simulink model "SSD_Pro"  (R2025b)
settings: Solver=FixedStepDiscrete  StartTime=0.0  StopTime=200  FixedStep=0.1  RelTol=1e-3
InitFcn:
  | addpath('C:\Users\dhanv\OneDrive\Desktop\ByteForce-Simulation\ByteForce-Simulation\simulink'); rehash;
undefined symbols (not defined in the file or in its folder): computeEventCode, DiscIntNeverNeededParam, simulinkPublishStep
libraries: simulink x6
settings Model: DataTypeOverride=Double  Creator=dhanv  LastModifiedBy=dhanv

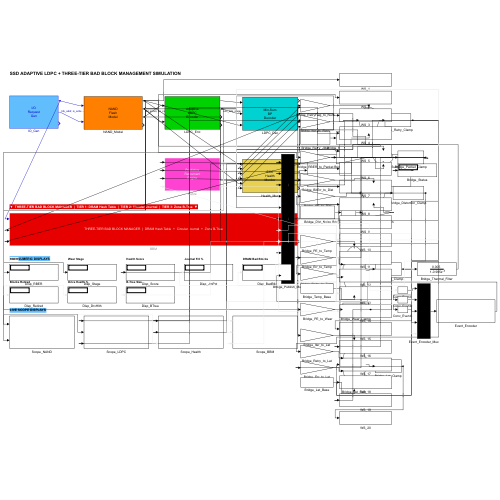
[thumbnail: Simulink's stored preview of the top-level diagram]
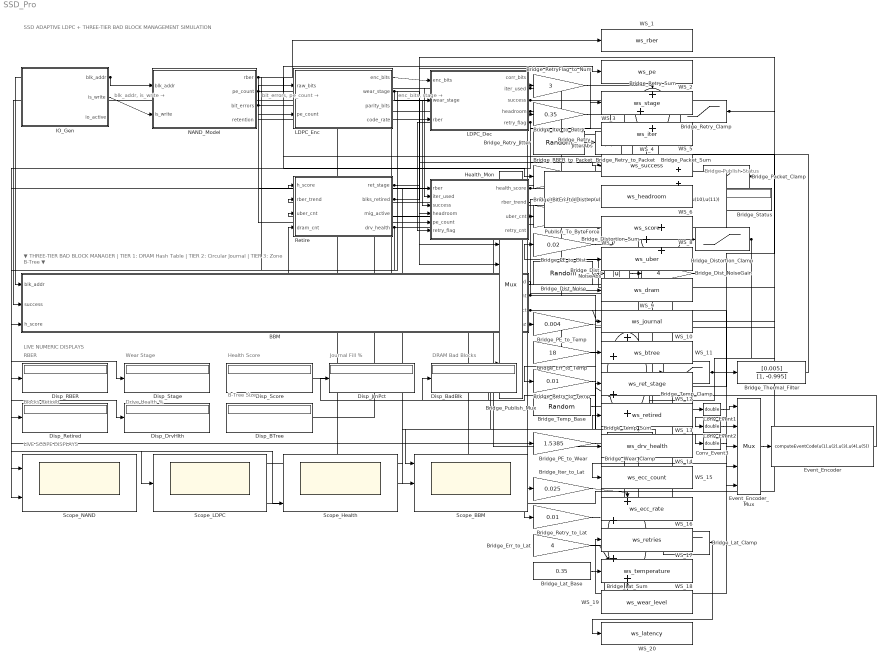
== system SSD_Pro ==
  note: Bridge Publish Status
  note: RBER
  note: Wear Stage
  note: Health Score
  note: Journal Fill %
  note: DRAM Bad Blocks
  note: Blocks Retired
  note: Drive Health %
  note: B-Tree Size
  note: blk_addr, is_write →
  note: bit_errors, pe_count →
  note: enc_bits, stage →
  note: SSD ADAPTIVE LDPC + THREE-TIER BAD BLOCK MANAGEMENT SIMULATION
  note: ▼ THREE-TIER BAD BLOCK MANAGER | TIER 1: DRAM Hash Table | TIER 2: Circular Journal | TIER 3: Zone B-Tree ▼
  note: LIVE NUMERIC DISPLAYS
  note: LIVE SCOPE DISPLAYS
  BBM : Subsystem
      mask Display: disp('THREE-TIER BAD BLOCK MANAGER  |  DRAM Hash Table  +  Circular Journal  +  Zone B-Tree')
  Bridge_BitErr_to_Dist : Gain  Gain=0.25
  Bridge_Dist_Noise : RandomNumber  Seed=9340  SampleTime=0.1
  Bridge_Dist_NoiseAbs : Abs  SaturateOnIntegerOverflow=off
  Bridge_Dist_NoiseGain : Gain  Gain=4
  Bridge_Distortion_Clamp : Saturate  UpperLimit=1e6  LowerLimit=0
  Bridge_Distortion_Sum : Sum  Inputs=+++
  Bridge_Err_to_Lat : Gain  Gain=4
  Bridge_Err_to_Temp : Gain  Gain=18
  Bridge_Iter_to_Lat : Gain  Gain=0.025
  Bridge_Iter_to_Retry : Gain  Gain=0.35
  Bridge_Lat_Base : Constant  Value=0.35
  Bridge_Lat_Clamp : Saturate  UpperLimit=20  LowerLimit=0.1
  Bridge_Lat_Sum : Sum  Inputs=++++
  Bridge_PE_to_Dist : Gain  Gain=0.02
  Bridge_PE_to_Temp : Gain  Gain=0.004
  Bridge_PE_to_Wear : Gain  Gain=1.5385
  Bridge_Packet_Clamp : Saturate  UpperLimit=1  LowerLimit=0
  Bridge_Packet_Sum : Sum
  Bridge_Publish_Mux : Mux  Inputs=11
  Bridge_RBER_to_Packet : Gain  Gain=4
  Bridge_RetryFlag_to_Num : Gain  Gain=3
  Bridge_Retry_Clamp : Saturate  UpperLimit=250  LowerLimit=0
  Bridge_Retry_Jitter : RandomNumber  Variance=4  Seed=8492  SampleTime=0.1
  Bridge_Retry_JitterAbs : Abs  SaturateOnIntegerOverflow=off
  Bridge_Retry_Sum : Sum  Inputs=+++
  Bridge_Retry_to_Lat : Gain  Gain=0.01
  Bridge_Retry_to_Packet : Gain  Gain=0.0015
  Bridge_Retry_to_Temp : Gain  Gain=0.01
  Bridge_Status : Display
  Bridge_Temp_Base : RandomNumber  Mean=30  Variance=25  Seed=6788  SampleTime=0.1
  Bridge_Temp_Clamp : Saturate  UpperLimit=95  LowerLimit=20
  Bridge_Temp_Sum : Sum  Inputs=++++
  Bridge_Thermal_Filter : DiscreteFilter  Numerator=[0.005]  Denominator=[1, -0.995]  SampleTime=0.1
  Bridge_Wear_Clamp : Saturate  UpperLimit=100  LowerLimit=0
  Conv_Event1 : DataTypeConversion  OutDataTypeStr=double  SaturateOnIntegerOverflow=off  RndMeth=Floor
  Conv_Event2 : DataTypeConversion  OutDataTypeStr=double  SaturateOnIntegerOverflow=off  RndMeth=Floor
  Conv_Event3 : DataTypeConversion  OutDataTypeStr=double  SaturateOnIntegerOverflow=off  RndMeth=Floor
  Disp_BTree : Display
  Disp_BadBlk : Display
  Disp_DrvHlth : Display
  Disp_JrnPct : Display
  Disp_RBER : Display
  Disp_Retired : Display
  Disp_Score : Display
  Disp_Stage : Display
  Event_Encoder : MATLABFcn  MATLABFcn=computeEventCode(u(1),u(2),u(3),u(4),u(5))
  Event_Encoder_Mux : Mux  Inputs=5
  Health_Mon : Subsystem
      mask Display: disp('ECC\nHealth\nMonitor')
  IO_Gen : Subsystem
      mask Display: disp('I/O\nRequest\nGen')
  LDPC_Dec : Subsystem
      mask Display: disp('Min-Sum\nBP\nDecoder')
  LDPC_Enc : Subsystem
      mask Display: disp('Adaptive\nLDPC\nEncoder')
  NAND_Model : Subsystem
      mask Display: disp('NAND\nFlash\nModel')
  Publish_To_ByteForce : MATLABFcn  MATLABFcn=simulinkPublishStep(u(1),u(2),u(3),u(4),u(5),u(6),u(7),u(8),u(9),u(10),u(11))
  Retire : Subsystem
      mask Display: disp('Predictive\nRetirement\nEngine')
  Scope_BBM : Scope  NumInputPorts=3
      settings: Title=Three-Tier BBM: DRAM Count | Journal % | B-Tree Size  YLabel=Count / %
  Scope_Health : Scope  NumInputPorts=3
      settings: Title=Block Health Score | UBER Count | Retirement Stage  YLabel=Value
  Scope_LDPC : Scope  NumInputPorts=3
      settings: Title=LDPC Decoder: Iterations | Success | Headroom %  YLabel=Value
  Scope_NAND : Scope  NumInputPorts=2
      settings: Title=NAND Degradation: RBER & PE Count  YLabel=Value
  WS_1 : ToWorkspace  VariableName=ws_rber  SaveFormat=Structure With Time  SampleTime=0.1
  WS_10 : ToWorkspace  VariableName=ws_journal  SaveFormat=Structure With Time  SampleTime=0.1
  WS_11 : ToWorkspace  VariableName=ws_btree  SaveFormat=Structure With Time  SampleTime=0.1
  WS_12 : ToWorkspace  VariableName=ws_ret_stage  SaveFormat=Structure With Time  SampleTime=0.1
  WS_13 : ToWorkspace  VariableName=ws_retired  SaveFormat=Structure With Time  SampleTime=0.1
  WS_14 : ToWorkspace  VariableName=ws_drv_health  SaveFormat=Structure With Time  SampleTime=0.1
  WS_15 : ToWorkspace  VariableName=ws_ecc_count  SaveFormat=Structure With Time  SampleTime=0.1
  WS_16 : ToWorkspace  VariableName=ws_ecc_rate  SaveFormat=Structure With Time  SampleTime=0.1
  WS_17 : ToWorkspace  VariableName=ws_retries  SaveFormat=Structure With Time  SampleTime=0.1
  WS_18 : ToWorkspace  VariableName=ws_temperature  SaveFormat=Structure With Time  SampleTime=0.1
  WS_19 : ToWorkspace  VariableName=ws_wear_level  SaveFormat=Structure With Time  SampleTime=0.1
  WS_2 : ToWorkspace  VariableName=ws_pe  SaveFormat=Structure With Time  SampleTime=0.1
  WS_20 : ToWorkspace  VariableName=ws_latency  SaveFormat=Structure With Time  SampleTime=0.1
  WS_3 : ToWorkspace  VariableName=ws_stage  SaveFormat=Structure With Time  SampleTime=0.1
  WS_4 : ToWorkspace  VariableName=ws_iter  SaveFormat=Structure With Time  SampleTime=0.1
  WS_5 : ToWorkspace  VariableName=ws_success  SaveFormat=Structure With Time  SampleTime=0.1
  WS_6 : ToWorkspace  VariableName=ws_headroom  SaveFormat=Structure With Time  SampleTime=0.1
  WS_7 : ToWorkspace  VariableName=ws_score  SaveFormat=Structure With Time  SampleTime=0.1
  WS_8 : ToWorkspace  VariableName=ws_uber  SaveFormat=Structure With Time  SampleTime=0.1
  WS_9 : ToWorkspace  VariableName=ws_dram  SaveFormat=Structure With Time  SampleTime=0.1
  wires:
  IO_Gen/1(blk_addr) -> NAND_Model/1(blk_addr), BBM/1(blk_addr)
  IO_Gen/2(is_write) -> NAND_Model/2(is_write)
  NAND_Model/3(bit_errors) -> LDPC_Enc/1(raw_bits), Bridge_BitErr_to_Dist/1
  NAND_Model/2(pe_count) -> LDPC_Enc/2(pe_count), Health_Mon/5(pe_count), Bridge_PE_to_Dist/1, Bridge_PE_to_Temp/1, Bridge_PE_to_Wear/1, Scope_NAND/2, WS_2/1
  LDPC_Enc/1(enc_bits) -> LDPC_Dec/1(enc_bits)
  LDPC_Enc/2(wear_stage) -> LDPC_Dec/2(wear_stage), Event_Encoder_Mux/4, Disp_Stage/1, WS_3/1
  NAND_Model/1(rber) -> LDPC_Dec/3(rber), Health_Mon/1(rber), Bridge_RBER_to_Packet/1, Disp_RBER/1, Scope_NAND/1, WS_1/1
  LDPC_Dec/2(iter_used) -> Health_Mon/2(iter_used), Bridge_Iter_to_Retry/1, Bridge_Iter_to_Lat/1, Scope_LDPC/1, WS_4/1
  LDPC_Dec/3(success) -> Health_Mon/3(success), BBM/2(success), Conv_Event2/1, Scope_LDPC/2, WS_5/1
  LDPC_Dec/4(headroom) -> Health_Mon/4(headroom), Scope_LDPC/3, WS_6/1
  LDPC_Dec/5(retry_flag) -> Health_Mon/6(retry_flag), Bridge_RetryFlag_to_Num/1, Conv_Event3/1
  Health_Mon/1(health_score) -> BBM/3(h_score), Retire/1(h_score), Disp_Score/1, Scope_Health/1, WS_7/1
  Health_Mon/2(rber_trend) -> Retire/2(rber_trend)
  Health_Mon/3(uber_cnt) -> Retire/3(uber_cnt), Bridge_Publish_Mux/9, Scope_Health/2, WS_8/1
  BBM/2(dram_cnt) -> Retire/4(dram_cnt), Bridge_Publish_Mux/7, Disp_BadBlk/1, Scope_BBM/1, WS_9/1
  Bridge_Retry_Jitter/1 -> Bridge_Retry_JitterAbs/1
  Bridge_RetryFlag_to_Num/1 -> Bridge_Retry_Sum/1
  Bridge_Iter_to_Retry/1 -> Bridge_Retry_Sum/2
  Bridge_Retry_JitterAbs/1 -> Bridge_Retry_Sum/3
  Bridge_Retry_Sum/1 -> Bridge_Retry_Clamp/1
  Bridge_Retry_Clamp/1 -> Bridge_Retry_to_Packet/1, Bridge_Retry_to_Temp/1, Bridge_Retry_to_Lat/1, Bridge_Publish_Mux/3, WS_17/1
  Bridge_RBER_to_Packet/1 -> Bridge_Packet_Sum/1
  Bridge_Retry_to_Packet/1 -> Bridge_Packet_Sum/2
  Bridge_Packet_Sum/1 -> Bridge_Packet_Clamp/1
  Bridge_Dist_Noise/1 -> Bridge_Dist_NoiseAbs/1
  Bridge_Dist_NoiseAbs/1 -> Bridge_Dist_NoiseGain/1
  Bridge_BitErr_to_Dist/1 -> Bridge_Distortion_Sum/1
  Bridge_PE_to_Dist/1 -> Bridge_Distortion_Sum/2
  Bridge_Dist_NoiseGain/1 -> Bridge_Distortion_Sum/3
  Bridge_Distortion_Sum/1 -> Bridge_Distortion_Clamp/1
  Bridge_Packet_Clamp/1 -> Bridge_Err_to_Temp/1, Bridge_Err_to_Lat/1, Bridge_Publish_Mux/2, WS_16/1
  Bridge_PE_to_Temp/1 -> Bridge_Temp_Sum/1
  Bridge_Err_to_Temp/1 -> Bridge_Temp_Sum/2
  Bridge_Retry_to_Temp/1 -> Bridge_Temp_Sum/3
  Bridge_Temp_Base/1 -> Bridge_Temp_Sum/4
  Bridge_Temp_Sum/1 -> Bridge_Temp_Clamp/1
  Bridge_PE_to_Wear/1 -> Bridge_Wear_Clamp/1
  Bridge_Iter_to_Lat/1 -> Bridge_Lat_Sum/1
  Bridge_Retry_to_Lat/1 -> Bridge_Lat_Sum/2
  Bridge_Err_to_Lat/1 -> Bridge_Lat_Sum/3
  Bridge_Lat_Base/1 -> Bridge_Lat_Sum/4
  Bridge_Lat_Sum/1 -> Bridge_Lat_Clamp/1
  Bridge_Temp_Clamp/1 -> Bridge_Thermal_Filter/1, WS_18/1
  BBM/1(is_bad) -> Conv_Event1/1
  Conv_Event1/1 -> Event_Encoder_Mux/1
  Conv_Event2/1 -> Event_Encoder_Mux/2
  Conv_Event3/1 -> Event_Encoder_Mux/3
  BBM/3(journal_pct) -> Event_Encoder_Mux/5, Bridge_Publish_Mux/8, Disp_JrnPct/1, Scope_BBM/2, WS_10/1
  Event_Encoder_Mux/1 -> Event_Encoder/1
  Event_Encoder/1 -> Bridge_Publish_Mux/11
  Bridge_Distortion_Clamp/1 -> Bridge_Publish_Mux/1, WS_15/1
  Bridge_Thermal_Filter/1 -> Bridge_Publish_Mux/4
  Bridge_Wear_Clamp/1 -> Bridge_Publish_Mux/5, WS_19/1
  Bridge_Lat_Clamp/1 -> Bridge_Publish_Mux/6, WS_20/1
  Retire/1(ret_stage) -> Bridge_Publish_Mux/10, Scope_Health/3, WS_12/1
  Bridge_Publish_Mux/1 -> Publish_To_ByteForce/1
  Publish_To_ByteForce/1 -> Bridge_Status/1
  Retire/2(blks_retired) -> Disp_Retired/1, WS_13/1
  Retire/4(drv_health) -> Disp_DrvHlth/1, WS_14/1
  BBM/4(btree_sz) -> Disp_BTree/1, Scope_BBM/3, WS_11/1

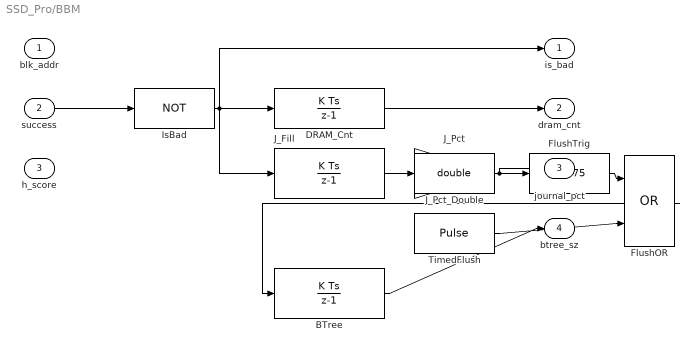
== system SSD_Pro/BBM ==
  blk_addr : Inport
  success : Inport  Port=2
  h_score : Inport  Port=3
  BTree : DiscreteIntegrator  SampleTime=0.1  UpperSaturationLimit=512  ICPrevOutput=DiscIntNeverNeededParam  ICPrevScaledInput=DiscIntNeverNeededParam
  DRAM_Cnt : DiscreteIntegrator  SampleTime=0.1  UpperSaturationLimit=512  ICPrevOutput=DiscIntNeverNeededParam  ICPrevScaledInput=DiscIntNeverNeededParam
  FlushOR : Logic  Operator=OR  AllPortsSameDT=off  OutDataTypeStr=boolean
  FlushTrig : simulink/Logic and Bit Operations/Compare To Constant  relop=>=  const=75  OutDataTypeStr=boolean
  IsBad : Logic  Operator=NOT  AllPortsSameDT=off  OutDataTypeStr=boolean
  J_Fill : DiscreteIntegrator  SampleTime=0.1  UpperSaturationLimit=64  LowerSaturationLimit=0  ICPrevOutput=DiscIntNeverNeededParam  ICPrevScaledInput=DiscIntNeverNeededParam
  J_Pct : Gain  Gain=1.5625
  J_Pct_Double : DataTypeConversion  OutDataTypeStr=double  RndMeth=Floor
  TimedFlush : DiscretePulseGenerator  PulseType=Time based  Period=15  PulseWidth=10
  is_bad : Outport
  dram_cnt : Outport  Port=2
  journal_pct : Outport  Port=3
  btree_sz : Outport  Port=4
  wires:
  success/1 -> IsBad/1
  IsBad/1 -> is_bad/1, DRAM_Cnt/1, J_Fill/1
  DRAM_Cnt/1 -> dram_cnt/1
  J_Fill/1 -> J_Pct/1
  J_Pct/1 -> journal_pct/1, J_Pct_Double/1
  J_Pct_Double/1 -> FlushTrig/1
  FlushTrig/1 -> FlushOR/1
  TimedFlush/1 -> FlushOR/2
  FlushOR/1 -> BTree/1
  BTree/1 -> btree_sz/1

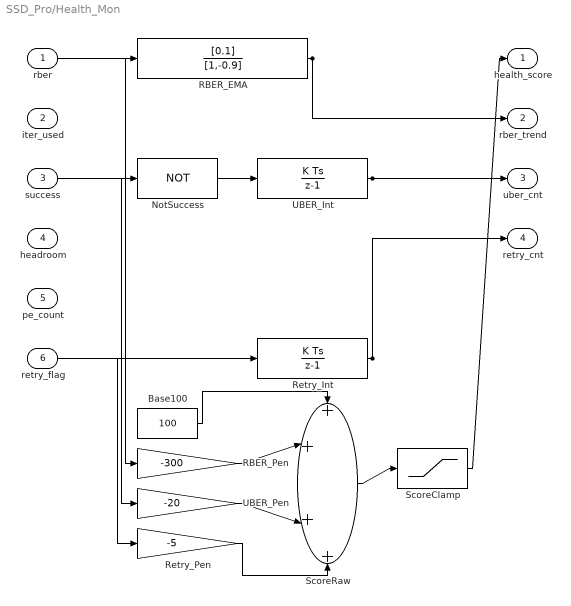
== system SSD_Pro/Health_Mon ==
  rber : Inport
  iter_used : Inport  Port=2
  success : Inport  Port=3
  headroom : Inport  Port=4
  pe_count : Inport  Port=5
  retry_flag : Inport  Port=6
  Base100 : Constant  Value=100
  NotSuccess : Logic  Operator=NOT  AllPortsSameDT=off  OutDataTypeStr=boolean
  RBER_EMA : DiscreteFilter  Numerator=[0.1]  Denominator=[1,-0.9]  SampleTime=0.1
  RBER_Pen : Gain  Gain=-300
  Retry_Int : DiscreteIntegrator  SampleTime=0.1  ICPrevOutput=DiscIntNeverNeededParam  ICPrevScaledInput=DiscIntNeverNeededParam
  Retry_Pen : Gain  Gain=-5
  ScoreClamp : Saturate  UpperLimit=100  LowerLimit=0
  ScoreRaw : Sum  Inputs=++++
  UBER_Int : DiscreteIntegrator  SampleTime=0.1  ICPrevOutput=DiscIntNeverNeededParam  ICPrevScaledInput=DiscIntNeverNeededParam
  UBER_Pen : Gain  Gain=-20
  health_score : Outport
  rber_trend : Outport  Port=2
  uber_cnt : Outport  Port=3
  retry_cnt : Outport  Port=4
  wires:
  rber/1 -> RBER_EMA/1
  RBER_EMA/1 -> rber_trend/1, RBER_Pen/1
  success/1 -> NotSuccess/1
  NotSuccess/1 -> UBER_Int/1
  UBER_Int/1 -> uber_cnt/1, UBER_Pen/1
  retry_flag/1 -> Retry_Int/1
  Retry_Int/1 -> retry_cnt/1, Retry_Pen/1
  Base100/1 -> ScoreRaw/1
  RBER_Pen/1 -> ScoreRaw/2
  UBER_Pen/1 -> ScoreRaw/3
  Retry_Pen/1 -> ScoreRaw/4
  ScoreRaw/1 -> ScoreClamp/1
  ScoreClamp/1 -> health_score/1

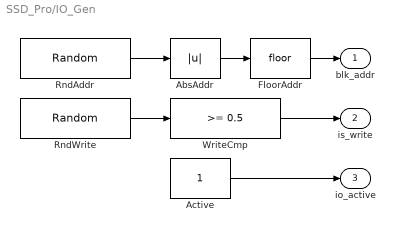
== system SSD_Pro/IO_Gen ==
  AbsAddr : Abs  SaturateOnIntegerOverflow=off
  Active : Constant
  FloorAddr : Rounding
  RndAddr : RandomNumber  Mean=256  Variance=29127.1111  Seed=6558  SampleTime=0.1
  RndWrite : RandomNumber  Mean=0.3  Variance=0.21  Seed=358  SampleTime=0.1
  WriteCmp : simulink/Logic and Bit Operations/Compare To Constant  relop=>=  const=0.5  OutDataTypeStr=boolean
  blk_addr : Outport
  is_write : Outport  Port=2
  io_active : Outport  Port=3
  wires:
  RndAddr/1 -> AbsAddr/1
  AbsAddr/1 -> FloorAddr/1
  FloorAddr/1 -> blk_addr/1
  RndWrite/1 -> WriteCmp/1
  WriteCmp/1 -> is_write/1
  Active/1 -> io_active/1

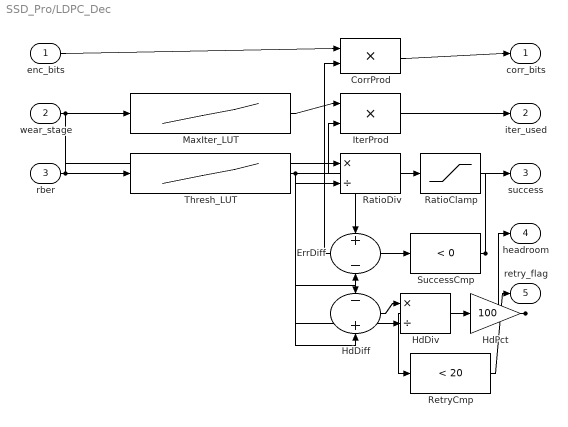
== system SSD_Pro/LDPC_Dec ==
  enc_bits : Inport
  wear_stage : Inport  Port=2
  rber : Inport  Port=3
  CorrProd : Product
  ErrDiff : Sum  Inputs=+-
  HdDiff : Sum  Inputs=-+
  HdDiv : Product  Inputs=*/
  HdPct : Gain  Gain=100
  IterProd : Product
  MaxIter_LUT : Lookup_n-D  NumberOfTableDimensions=1  BreakpointsForDimension1=[1,2,3,4]  Table=[10,20,50,100]  InternalRulePriority=Speed  RndMeth=Simplest
  RatioClamp : Saturate  UpperLimit=1  LowerLimit=0
  RatioDiv : Product  Inputs=*/
  RetryCmp : simulink/Logic and Bit Operations/Compare To Constant  relop=<  const=20  OutDataTypeStr=boolean
  SuccessCmp : simulink/Logic and Bit Operations/Compare To Zero  relop=<  OutDataTypeStr=boolean
  Thresh_LUT : Lookup_n-D  NumberOfTableDimensions=1  BreakpointsForDimension1=[1,2,3,4]  Table=[0.020000,0.100000,0.500000,1.000000]  InternalRulePriority=Speed  RndMeth=Simplest
  corr_bits : Outport
  iter_used : Outport  Port=2
  success : Outport  Port=3
  headroom : Outport  Port=4
  retry_flag : Outport  Port=5
  wires:
  wear_stage/1 -> MaxIter_LUT/1, Thresh_LUT/1
  rber/1 -> RatioDiv/1, ErrDiff/1, HdDiff/1
  Thresh_LUT/1 -> RatioDiv/2, ErrDiff/2, HdDiff/2, HdDiv/2
  RatioDiv/1 -> RatioClamp/1
  MaxIter_LUT/1 -> IterProd/1
  RatioClamp/1 -> IterProd/2
  IterProd/1 -> iter_used/1
  ErrDiff/1 -> SuccessCmp/1
  SuccessCmp/1 -> success/1, CorrProd/2
  HdDiff/1 -> HdDiv/1
  HdDiv/1 -> HdPct/1
  HdPct/1 -> headroom/1, RetryCmp/1
  RetryCmp/1 -> retry_flag/1
  enc_bits/1 -> CorrProd/1
  CorrProd/1 -> corr_bits/1

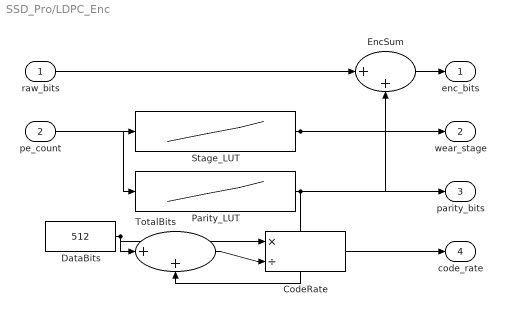
== system SSD_Pro/LDPC_Enc ==
  raw_bits : Inport
  pe_count : Inport  Port=2
  CodeRate : Product  Inputs=*/
  DataBits : Constant  Value=512
  EncSum : Sum  Inputs=|++
  Parity_LUT : Lookup_n-D  NumberOfTableDimensions=1  BreakpointsForDimension1=[1, 2, 3, 4]  Table=[10,20,40,100]  InternalRulePriority=Speed  RndMeth=Simplest
  Stage_LUT : Lookup_n-D  NumberOfTableDimensions=1  BreakpointsForDimension1=[0, 16, 33, 49]  Table=[1, 2, 3, 4]  InternalRulePriority=Speed  RndMeth=Simplest
  TotalBits : Sum  Inputs=|++
  enc_bits : Outport
  wear_stage : Outport  Port=2
  parity_bits : Outport  Port=3
  code_rate : Outport  Port=4
  wires:
  pe_count/1 -> Stage_LUT/1
  Stage_LUT/1 -> wear_stage/1, Parity_LUT/1
  Parity_LUT/1 -> parity_bits/1, EncSum/2, TotalBits/2
  raw_bits/1 -> EncSum/1
  EncSum/1 -> enc_bits/1
  DataBits/1 -> TotalBits/1, CodeRate/1
  TotalBits/1 -> CodeRate/2
  CodeRate/1 -> code_rate/1

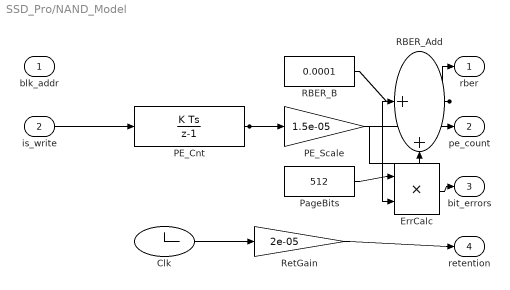
== system SSD_Pro/NAND_Model ==
  blk_addr : Inport
  is_write : Inport  Port=2
  Clk : Clock
  ErrCalc : Product
  PE_Cnt : DiscreteIntegrator  SampleTime=0.1  UpperSaturationLimit=65  ICPrevOutput=DiscIntNeverNeededParam  ICPrevScaledInput=DiscIntNeverNeededParam
  PE_Scale : Gain  Gain=1.5e-05
  PageBits : Constant  Value=512
  RBER_Add : Sum  Inputs=|++
  RBER_B : Constant  Value=0.0001
  RetGain : Gain  Gain=2e-05
  rber : Outport
  pe_count : Outport  Port=2
  bit_errors : Outport  Port=3
  retention : Outport  Port=4
  wires:
  is_write/1 -> PE_Cnt/1
  PE_Cnt/1 -> pe_count/1, PE_Scale/1
  RBER_B/1 -> RBER_Add/1
  PE_Scale/1 -> RBER_Add/2
  RBER_Add/1 -> rber/1, ErrCalc/2
  PageBits/1 -> ErrCalc/1
  ErrCalc/1 -> bit_errors/1
  Clk/1 -> RetGain/1
  RetGain/1 -> retention/1

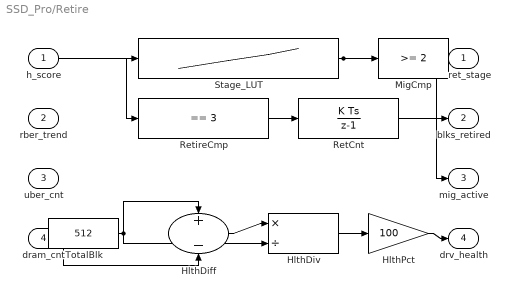
== system SSD_Pro/Retire ==
  h_score : Inport
  rber_trend : Inport  Port=2
  uber_cnt : Inport  Port=3
  dram_cnt : Inport  Port=4
  HlthDiff : Sum  Inputs=+-
  HlthDiv : Product  Inputs=*/
  HlthPct : Gain  Gain=100
  MigCmp : simulink/Logic and Bit Operations/Compare To Constant  relop=>=  const=2  OutDataTypeStr=boolean
  RetCnt : DiscreteIntegrator  SampleTime=0.1  UpperSaturationLimit=512  ICPrevOutput=DiscIntNeverNeededParam  ICPrevScaledInput=DiscIntNeverNeededParam
  RetireCmp : simulink/Logic and Bit Operations/Compare To Constant  relop===  const=3  OutDataTypeStr=boolean
  Stage_LUT : Lookup_n-D  NumberOfTableDimensions=1  BreakpointsForDimension1=[0,20,50,70,100]  Table=[3,3,2,1,0]  InternalRulePriority=Speed  RndMeth=Simplest
  TotalBlk : Constant  Value=512
  ret_stage : Outport
  blks_retired : Outport  Port=2
  mig_active : Outport  Port=3
  drv_health : Outport  Port=4
  wires:
  h_score/1 -> Stage_LUT/1
  Stage_LUT/1 -> ret_stage/1, MigCmp/1, RetireCmp/1
  MigCmp/1 -> mig_active/1
  RetireCmp/1 -> RetCnt/1
  RetCnt/1 -> blks_retired/1
  TotalBlk/1 -> HlthDiff/1, HlthDiv/2
  dram_cnt/1 -> HlthDiff/2
  HlthDiff/1 -> HlthDiv/1
  HlthDiv/1 -> HlthPct/1
  HlthPct/1 -> drv_health/1
